simulink model "teleoperation_no_two_layer"  (R2020a)
settings: Solver=VariableStepAuto  StartTime=0.0  StopTime=7  RelTol=1e-3
values from neighbouring files (symbols this model uses):
  B = 1 / k_m    (= 0.0517063081696)    [Teleop_parameters.m]    (also in base.mat; base_no_attrito.mat = 0; ci_siamo.mat; force_control.mat)
  Be = 0.5    [Teleop_parameters.m]    (also in base.mat; base_no_attrito.mat; ci_siamo.mat = 5; force_control.mat)
  Bh = 0.02    [Teleop_parameters.m]    (also in base.mat; base_no_attrito.mat; ci_siamo.mat; force_control.mat)
  Fc_h = 5    [Teleop_parameters.m]    (also in base.mat; base_no_attrito.mat; ci_siamo.mat; force_control.mat)
  J = tau_m / k_m    (= 0.0629265770424)    [Teleop_parameters.m]    (also in base.mat; base_no_attrito.mat; ci_siamo.mat; force_control.mat)
  J_r = J + 0.5 * J    (= 0.0943898655636)    [Teleop_parameters.m]    (also in base.mat; base_no_attrito.mat; ci_siamo.mat = 0.0629265770424; force_control.mat)
  Jh = 0.02    [Teleop_parameters.m]    (also in base.mat; base_no_attrito.mat; ci_siamo.mat; force_control.mat)
  Kc2v_m = 2    [Teleop_parameters.m]    (also in base.mat; base_no_attrito.mat; ci_siamo.mat; force_control.mat)
  Kc2v_s = 2    [Teleop_parameters.m]    (also in base.mat; base_no_attrito.mat; ci_siamo.mat; force_control.mat)
  Kd_h = 1    [Teleop_parameters.m]    (also in base.mat; base_no_attrito.mat; ci_siamo.mat = 10; force_control.mat)
  Kd_m = 1    [Teleop_parameters.m]    (also in base.mat; base_no_attrito.mat; ci_siamo.mat = 0.005; force_control.mat)
  Kd_s = 1    [Teleop_parameters.m]    (also in base.mat; base_no_attrito.mat; ci_siamo.mat = 0.5; force_control.mat)
  Ke = 10    [Teleop_parameters.m]    (also in base.mat; base_no_attrito.mat; ci_siamo.mat; force_control.mat)
  Kp_h = 1.2    [Teleop_parameters.m]    (also in base.mat; base_no_attrito.mat; ci_siamo.mat = 10; force_control.mat)
  Kp_m = 1    [Teleop_parameters.m]    (also in base.mat; base_no_attrito.mat; ci_siamo.mat = 0.01; force_control.mat)
  Kp_s = 1    [Teleop_parameters.m]    (also in base.mat; base_no_attrito.mat; ci_siamo.mat; force_control.mat)
  Kt2c_m = 1.182    [Teleop_parameters.m]    (also in base.mat; base_no_attrito.mat; ci_siamo.mat; force_control.mat)
  Kt2c_s = 1.182    [Teleop_parameters.m]    (also in base.mat; base_no_attrito.mat; ci_siamo.mat; force_control.mat)
  Kv_fc = 20    [Teleop_parameters.m]    (also in base.mat = 0; base_no_attrito.mat = 0; ci_siamo.mat = 10; force_control.mat = 30)
  lArm_m = 0.1    [Teleop_parameters.m]    (also in base.mat; base_no_attrito.mat; ci_siamo.mat; force_control.mat)
  lArm_s = 0.1    [Teleop_parameters.m]    (also in base.mat; base_no_attrito.mat; ci_siamo.mat; force_control.mat)
  qe = 0.5    [Teleop_parameters.m]    (also in base.mat = 5; base_no_attrito.mat = 5; ci_siamo.mat; force_control.mat = 5)
  Ts = 0.002    [Teleop_parameters.m]    (also in base.mat; base_no_attrito.mat; ci_siamo.mat; force_control.mat)
settings Model: Creator=gbagolin  LastModifiedBy=giova

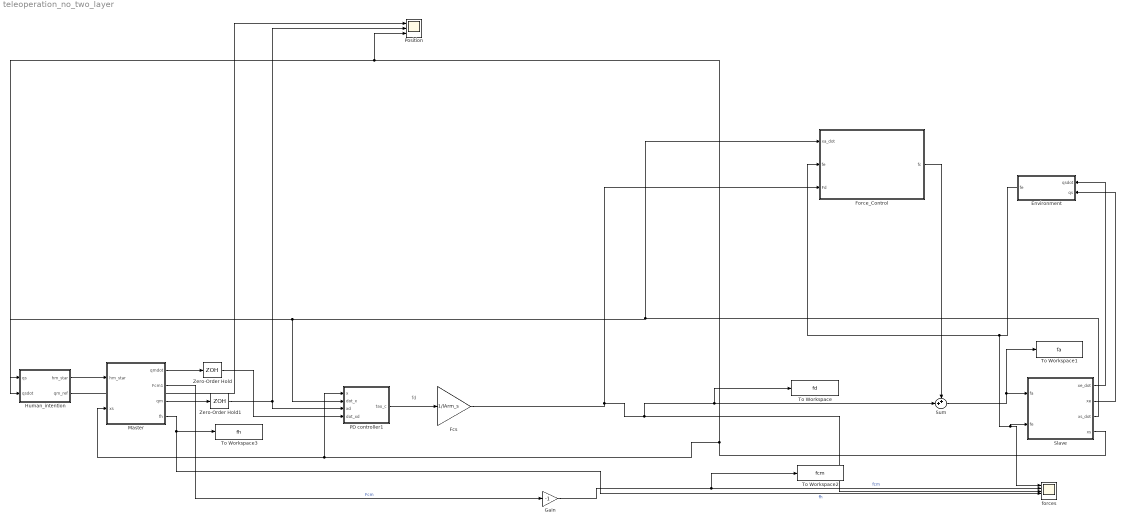
== system teleoperation_no_two_layer ==
  note: fd
  Environment : Subsystem
  Fcs : Gain  Gain=1/lArm_s
  Force_Control : Subsystem
  Gain : Gain  Gain=-1
  Human_intention : Subsystem
  Master : Subsystem
  PD controller1 : Subsystem
  Position : Scope  NumInputPorts=3
  Slave : Subsystem
  Sum : Sum  Inputs=++|
  To Workspace : ToWorkspace  VariableName=fd  SaveFormat=Timeseries  SampleTime=-1
  To Workspace1 : ToWorkspace  VariableName=fa  SaveFormat=Timeseries  SampleTime=-1
  To Workspace2 : ToWorkspace  VariableName=fcm  SaveFormat=Timeseries  SampleTime=-1
  To Workspace3 : ToWorkspace  VariableName=fh  SaveFormat=Timeseries  SampleTime=-1
  Zero-Order Hold : ZeroOrderHold  SampleTime=Ts
  Zero-Order Hold1 : ZeroOrderHold  SampleTime=Ts
  forces : Scope  NumInputPorts=5
  wires:
  Human_intention/1(hm_star) -> Master/1(hm_star)
  Sum/1 -> To Workspace1/1, Slave/1(fa)
  Master/2(Fcm1) -> Gain/1  "Fcm"
  Slave/1(xe_dot) -> Environment/1(qsdot)
  Slave/2(xe) -> Environment/2(qs)
  PD controller1/1(tau_c) -> Fcs/1
  Master/1(qmdot) -> Zero-Order Hold/1
  Human_intention/2(qm_ref) -> Position/1
  Master/4(fh) -> forces/4, To Workspace3/1  "fh"
  Gain/1 -> forces/2, To Workspace2/1  "fcm"
  Master/3(qm) -> Zero-Order Hold1/1
  Environment/1(fe) -> Force_Control/2(fe), forces/1, Slave/2(fe)
  Fcs/1 -> Force_Control/3(Fd), forces/3, Sum/2, To Workspace/1
  Force_Control/1(fc) -> Sum/1
  Zero-Order Hold/1 -> PD controller1/4(dot_xd)
  Zero-Order Hold1/1 -> Position/2, PD controller1/3(xd)
  Slave/4(xs) -> Master/2(xs), PD controller1/1(x), Human_intention/1(qs), Position/3
  Slave/3(xs_dot) -> Human_intention/2(qsdot), PD controller1/2(dot_x), Force_Control/1(xa_dot)

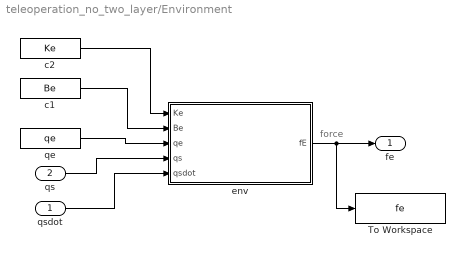
== system teleoperation_no_two_layer/Environment ==
  note: force
  qsdot : Inport
  qs : Inport  Port=2
  To Workspace : ToWorkspace  VariableName=fe  SaveFormat=Timeseries  SampleTime=-1
  c1 : Constant  Value=Be  SampleTime=0
  c2 : Constant  Value=Ke  SampleTime=0
  env : MATLAB Function  TreatAsAtomicUnit=on
  qe : Constant  Value=qe  SampleTime=0
  fe : Outport  VectorParamsAs1DForOutWhenUnconnected=off
  wires:
  qe/1 -> env/3(qe)
  c1/1 -> env/2(Be)
  c2/1 -> env/1(Ke)
  qs/1 -> env/4(qs)
  qsdot/1 -> env/5(qsdot)
  env/1(fE) -> To Workspace/1, fe/1

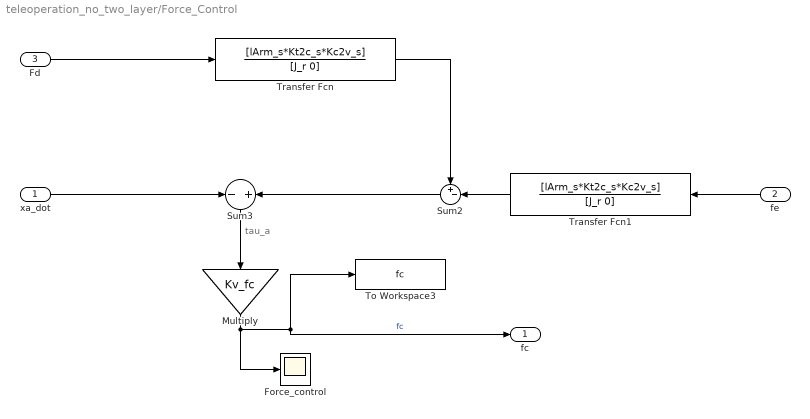
== system teleoperation_no_two_layer/Force_Control ==
  note: tau_a
  xa_dot : Inport
  fe : Inport  Port=2
  Fd : Inport  Port=3
  Force_control : Scope
  Multiply : Gain  Gain=Kv_fc
  Sum2 : Sum  Inputs=+-|
  Sum3 : Sum  Inputs=-|+
  To Workspace3 : ToWorkspace  VariableName=fc  SaveFormat=Timeseries  SampleTime=-1
  Transfer Fcn : TransferFcn  Numerator=[lArm_s*Kt2c_s*Kc2v_s]  Denominator=[J_r 0]
  Transfer Fcn1 : TransferFcn  Numerator=[lArm_s*Kt2c_s*Kc2v_s]  Denominator=[J_r 0]
  fc : Outport
  wires:
  Fd/1 -> Transfer Fcn/1
  Multiply/1 -> fc/1, To Workspace3/1, Force_control/1  "fc"
  Transfer Fcn1/1 -> Sum2/2
  Transfer Fcn/1 -> Sum2/1
  fe/1 -> Transfer Fcn1/1
  Sum2/1 -> Sum3/2
  Sum3/1 -> Multiply/1
  xa_dot/1 -> Sum3/1

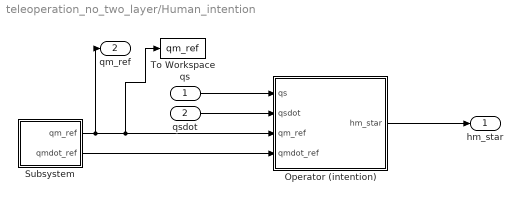
== system teleoperation_no_two_layer/Human_intention ==
  qs : Inport
  qsdot : Inport  Port=2
  Operator (intention) : Subsystem
  Subsystem : Subsystem
  To Workspace : ToWorkspace  VariableName=qm_ref  SaveFormat=Timeseries  SampleTime=-1
  hm_star : Outport
  qm_ref : Outport  Port=2
  wires:
  Subsystem/1(qm_ref) -> To Workspace/1, Operator (intention)/3(qm_ref), qm_ref/1
  Subsystem/2(qmdot_ref) -> Operator (intention)/4(qmdot_ref)
  Operator (intention)/1(hm_star) -> hm_star/1
  qs/1 -> Operator (intention)/1(qs)
  qsdot/1 -> Operator (intention)/2(qsdot)

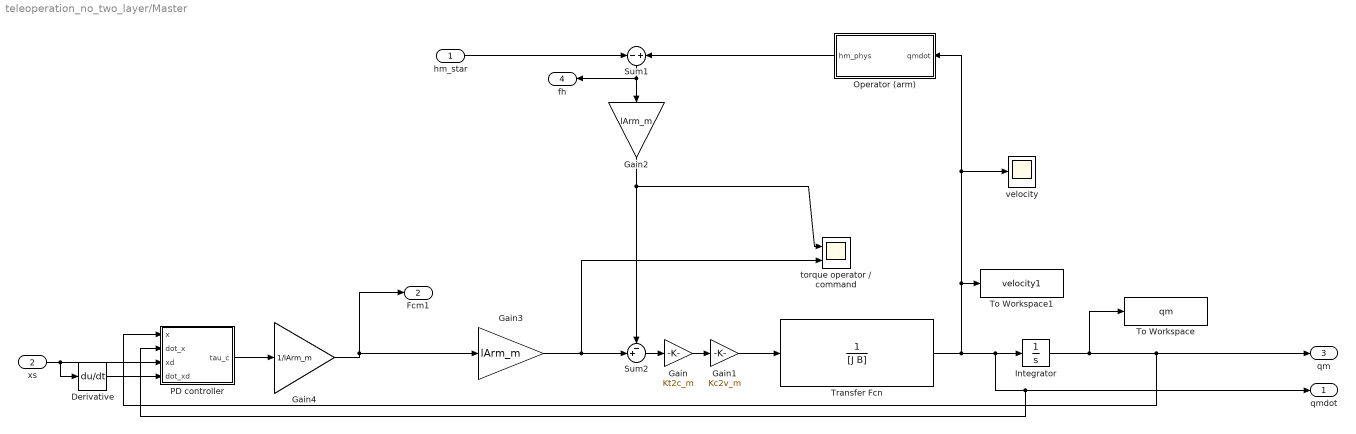
== system teleoperation_no_two_layer/Master ==
  hm_star : Inport
  xs : Inport  Port=2
  Derivative : Derivative
  Gain : Gain  Gain=Kt2c_m
  Gain1 : Gain  Gain=Kc2v_m
  Gain2 : Gain  Gain=lArm_m
  Gain3 : Gain  Gain=lArm_m
  Gain4 : Gain  Gain=1/lArm_m
  Integrator : Integrator
  Operator (arm) : Subsystem
  PD controller : Subsystem
  Sum1 : Sum  Inputs=-+
  Sum2 : Sum  Inputs=-+|
  To Workspace : ToWorkspace  VariableName=qm  SaveFormat=Timeseries  SampleTime=-1
  To Workspace1 : ToWorkspace  VariableName=velocity1  SaveFormat=Timeseries  SampleTime=-1
  Transfer Fcn : TransferFcn  Denominator=[J B]
  torque operator / command : Scope  NumInputPorts=2
  velocity : Scope
  qmdot : Outport
  Fcm1 : Outport  Port=2
  qm : Outport  Port=3
  fh : Outport  Port=4
  wires:
  Integrator/1 -> To Workspace/1, PD controller/1(x), qm/1
  Operator (arm)/1(hm_phys) -> Sum1/2
  Sum1/1 -> Gain2/1, fh/1
  Gain4/1 -> Fcm1/1, Gain3/1
  Transfer Fcn/1 -> Operator (arm)/1(qmdot), velocity/1, To Workspace1/1, PD controller/2(dot_x), qmdot/1, Integrator/1
  hm_star/1 -> Sum1/1
  Sum2/1 -> Gain/1
  Gain/1 -> Gain1/1
  Gain1/1 -> Transfer Fcn/1
  Gain2/1 -> torque operator / command/1, Sum2/1
  Gain3/1 -> torque operator / command/2, Sum2/2
  Derivative/1 -> PD controller/4(dot_xd)
  xs/1 -> Derivative/1, PD controller/3(xd)
  PD controller/1(tau_c) -> Gain4/1

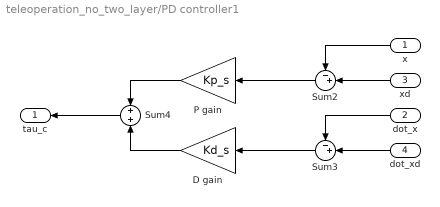
== system teleoperation_no_two_layer/PD controller1 ==
  x : Inport
  dot_x : Inport  Port=2
  xd : Inport  Port=3
  dot_xd : Inport  Port=4
  D gain : Gain  Gain=Kd_s
  P gain : Gain  Gain=Kp_s
  Sum2 : Sum  Inputs=-+|
  Sum3 : Sum  Inputs=-+|
  Sum4 : Sum
  tau_c : Outport  VectorParamsAs1DForOutWhenUnconnected=off
  wires:
  D gain/1 -> Sum4/2
  dot_x/1 -> Sum3/1
  dot_xd/1 -> Sum3/2
  x/1 -> Sum2/1
  xd/1 -> Sum2/2
  Sum3/1 -> D gain/1
  P gain/1 -> Sum4/1
  Sum4/1 -> tau_c/1
  Sum2/1 -> P gain/1

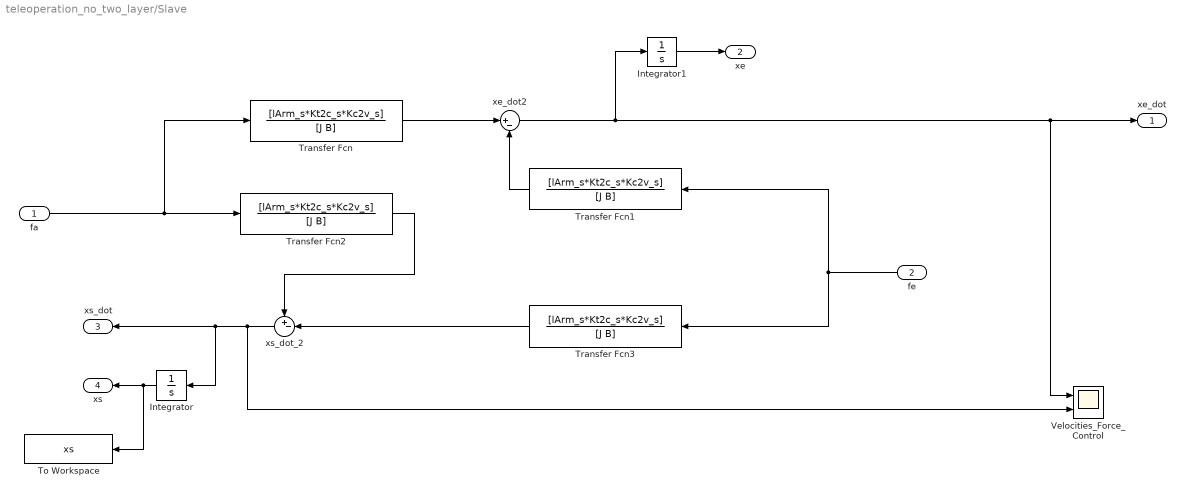
== system teleoperation_no_two_layer/Slave ==
  fa : Inport
  fe : Inport  Port=2
  Integrator : Integrator
  Integrator1 : Integrator
  To Workspace : ToWorkspace  VariableName=xs  SaveFormat=Timeseries  SampleTime=-1
  Transfer Fcn{,1..3} (4 alike) : TransferFcn  Numerator=[lArm_s*Kt2c_s*Kc2v_s]  Denominator=[J B]
  Velocities_Force_Control : Scope  NumInputPorts=2
  xe_dot2 : Sum  Inputs=|+-
  xs_dot_2 : Sum  Inputs=+-|
  xe_dot : Outport
  xe : Outport  Port=2
  xs_dot : Outport  Port=3
  xs : Outport  Port=4
  wires:
  fa/1 -> Transfer Fcn2/1, Transfer Fcn/1
  Transfer Fcn/1 -> xe_dot2/1
  xe_dot2/1 -> Integrator1/1, xe_dot/1, Velocities_Force_Control/1
  Transfer Fcn1/1 -> xe_dot2/2
  Transfer Fcn3/1 -> xs_dot_2/2
  Transfer Fcn2/1 -> xs_dot_2/1
  xs_dot_2/1 -> Velocities_Force_Control/2, Integrator/1, xs_dot/1
  fe/1 -> Transfer Fcn1/1, Transfer Fcn3/1
  Integrator/1 -> To Workspace/1, xs/1
  Integrator1/1 -> xe/1

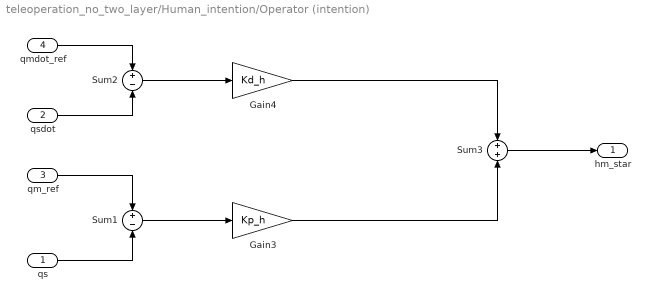
== system teleoperation_no_two_layer/Human_intention/Operator (intention) ==
  qs : Inport
  qsdot : Inport  Port=2
  qm_ref : Inport  Port=3
  qmdot_ref : Inport  Port=4
  Gain3 : Gain  Gain=Kp_h
  Gain4 : Gain  Gain=Kd_h
  Sum1 : Sum  Inputs=+|-
  Sum2 : Sum  Inputs=+|-
  Sum3 : Sum  Inputs=+|+
  hm_star : Outport  VectorParamsAs1DForOutWhenUnconnected=off
  wires:
  qs/1 -> Sum1/2
  qm_ref/1 -> Sum1/1
  qmdot_ref/1 -> Sum2/1
  Sum1/1 -> Gain3/1
  qsdot/1 -> Sum2/2
  Sum2/1 -> Gain4/1
  Gain4/1 -> Sum3/1
  Gain3/1 -> Sum3/2
  Sum3/1 -> hm_star/1

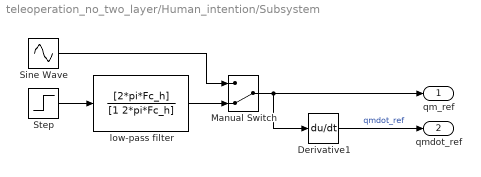
== system teleoperation_no_two_layer/Human_intention/Subsystem ==
  Derivative1 : Derivative  CoefficientInTFapproximation=0.001
  Manual Switch : ManualSwitch  CurrentSetting=0
  Sine Wave : Sin  SampleTime=0
  Step : Step  SampleTime=0
  low-pass filter : TransferFcn  Numerator=[2*pi*Fc_h]  Denominator=[1 2*pi*Fc_h]
  qm_ref : Outport
  qmdot_ref : Outport  Port=2
  wires:
  low-pass filter/1 -> Manual Switch/2
  Manual Switch/1 -> qm_ref/1, Derivative1/1
  Derivative1/1 -> qmdot_ref/1  "qmdot_ref"
  Step/1 -> low-pass filter/1
  Sine Wave/1 -> Manual Switch/1

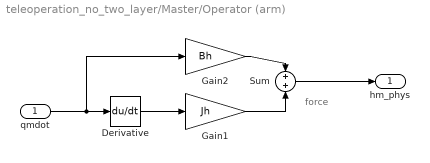
== system teleoperation_no_two_layer/Master/Operator (arm) ==
  note: force
  qmdot : Inport
  Derivative : Derivative  CoefficientInTFapproximation=0.001
  Gain1 : Gain  Gain=Jh
  Gain2 : Gain  Gain=Bh
  Sum : Sum  Inputs=+|+
  hm_phys : Outport  VectorParamsAs1DForOutWhenUnconnected=off
  wires:
  qmdot/1 -> Gain2/1, Derivative/1
  Sum/1 -> hm_phys/1
  Derivative/1 -> Gain1/1
  Gain2/1 -> Sum/1
  Gain1/1 -> Sum/2

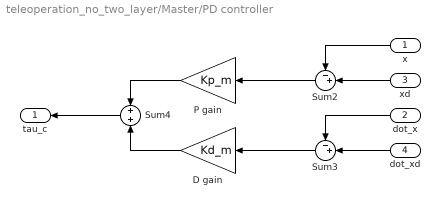
== system teleoperation_no_two_layer/Master/PD controller ==
  x : Inport
  dot_x : Inport  Port=2
  xd : Inport  Port=3
  dot_xd : Inport  Port=4
  D gain : Gain  Gain=Kd_m
  P gain : Gain  Gain=Kp_m
  Sum2 : Sum  Inputs=-+|
  Sum3 : Sum  Inputs=-+|
  Sum4 : Sum
  tau_c : Outport  VectorParamsAs1DForOutWhenUnconnected=off
  wires:
  D gain/1 -> Sum4/2
  dot_x/1 -> Sum3/1
  dot_xd/1 -> Sum3/2
  x/1 -> Sum2/1
  xd/1 -> Sum2/2
  Sum3/1 -> D gain/1
  P gain/1 -> Sum4/1
  Sum4/1 -> tau_c/1
  Sum2/1 -> P gain/1

== matlab function teleoperation_no_two_layer/Environment/env ==
  data: Ke input; Be input; qe input; qs input; fE output; qsdot input
function fE  = environment(Ke, Be, qe, qs, qsdot)
if qs > qe
   fE = Ke * (qs - qe) + Be * qsdot;
else
   fE = 0;
end
